simulink model "kh4_controller"  (R2018a)
settings: Solver=ode15s  StartTime=0.0  StopTime=10.0  RelTol=1e-3
libraries: slctrlblks x2, dspinverses x1, simulink x1
settings Model: Creator=FlightControlLab  LastModifiedBy=FlightControlLab
settings SolverCC: SolverResetMethod=Robust

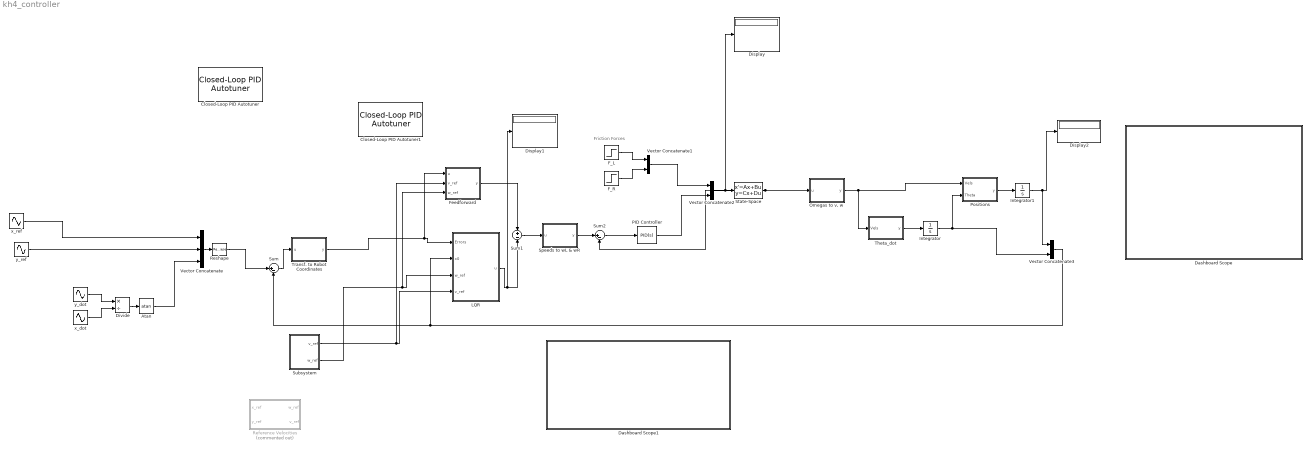
== system kh4_controller ==
  note: Friction Forces
  Atan : Trigonometry  Operator=atan
  Closed-Loop PID Autotuner : slctrlblks/Closed-Loop PID Autotuner  PIDType=PI  PIDForm=Parallel  TimeDomain=continuous-time  DiscreteTs=0.1  IntegratorFormula=Forward Euler  FilterFormula=Forward Euler  ContinuousTs=0.02  Bandwidth=1  UseExternalWC=off  TargetPM=60  UseExternalPM=off  UseExternalAchievedPM=off  PlantType=Stable  PlantSign=Positive  AmpSine=1  UseExternalAmpSine=off  UseExternalFRD=off  UseExternalU0=off  UseCompanion=off  NotDeployTuningModule=off  UsePLCCoder=off  BlockDataType=double  UseConnectedPID=on  blockpath=[]  tunedP=0  tunedI=0  tunedD=0  tunedN=100  tunedPM=0  EstimationWindowSize=3
      settings: SourceProductName=Simulink Control Design  SourceProductBaseCode=SD
  Closed-Loop PID Autotuner1 : slctrlblks/Closed-Loop PID Autotuner  PIDType=PI  PIDForm=Parallel  TimeDomain=discrete-time  DiscreteTs=0.1  IntegratorFormula=Forward Euler  FilterFormula=Forward Euler  ContinuousTs=0.02  Bandwidth=1  UseExternalWC=off  TargetPM=60  UseExternalPM=off  UseExternalAchievedPM=off  PlantType=Stable  PlantSign=Positive  AmpSine=1  UseExternalAmpSine=off  UseExternalFRD=off  UseExternalU0=off  UseCompanion=off  NotDeployTuningModule=off  UsePLCCoder=off  BlockDataType=double  UseConnectedPID=on  blockpath=[]  tunedP=0  tunedI=0  tunedD=0  tunedN=100  tunedPM=0  EstimationWindowSize=3
      settings: SourceProductName=Simulink Control Design  SourceProductBaseCode=SD
  Dashboard Scope : Subsystem  DialogController=hmiCreateDDGDialog  IsWebBlock=on  mask(MWDashboardBlock){webBlockId=dffbf5dc-94e7-4540-87c2-f2341032f13a, webBlockType=sdiscope, ShowInitialText=on, HMISrcModelName=kh4_controller}
      mask prompts: webBlockId "WebBlock Id"; webBlockType "WebBlock Type"; HMISrcModelName "Source Model"
      mask help: SimulinkHMI:dialogs:HMIScopeDialogDesc
      mask Help: helpview([docroot '/mapfiles/simulink.map'], 'hmi_scope')
      mask Display:
      | if strcmp(get_param(bdroot(gcb),'BlockDiagramType'), 'library')
      |     image([(matlabroot) '/toolbox/simulink/hmi/icons/DashboardScope.png']);
      | end
  Dashboard Scope1 : Subsystem  DialogController=hmiCreateDDGDialog  IsWebBlock=on  mask(MWDashboardBlock){webBlockId=52e07cf3-ffb0-4692-b96f-0b5126ad5948, webBlockType=sdiscope, ShowInitialText=on, HMISrcModelName=kh4_controller}
      mask prompts: webBlockId "WebBlock Id"; webBlockType "WebBlock Type"; HMISrcModelName "Source Model"
      mask help: SimulinkHMI:dialogs:HMIScopeDialogDesc
      mask Help: helpview([docroot '/mapfiles/simulink.map'], 'hmi_scope')
      mask Display:
      | if strcmp(get_param(bdroot(gcb),'BlockDiagramType'), 'library')
      |     image([(matlabroot) '/toolbox/simulink/hmi/icons/DashboardScope.png']);
      | end
  Display : Display
  Display1 : Display
  Display2 : Display
  Divide : Product  Inputs=*/
  F_L : Step  After=0.1  SampleTime=0
  F_R : Step  After=0.1  SampleTime=0
  Feedforward : MATLAB Function  TreatAsAtomicUnit=on
  Integrator : Integrator
  Integrator1 : Integrator
  LQR : Subsystem
  "Omegas to v, w" : MATLAB Function  TreatAsAtomicUnit=on
  PID Controller : simulink/Continuous/PID Controller  Controller=PID  TimeDomain=Continuous-time  SampleTime=-1  IntegratorMethod=Forward Euler  FilterMethod=Forward Euler  Form=Parallel  UseFilter=on  ControllerParametersSource=internal  P=10  I=10  D=1  N=100  InitialConditionSource=internal  InitialConditionForIntegrator=0  InitialConditionForFilter=0  ExternalReset=none  LimitOutput=off  UpperSaturationLimit=inf  LowerSaturationLimit=-inf  LinearizeAsGain=on  AntiWindupMode=none  Kb=1  TrackingMode=off  Kt=1  PParamMin=[]  PParamMax=[]  IParamMin=[]  IParamMax=[]  DParamMin=[]  DParamMax=[]  NParamMin=[]  NParamMax=[]  KbParamMin=[]  KbParamMax=[]  KtParamMin=[]  KtParamMax=[]  POutMin=[]  POutMax=[]  IOutMin=[]  IOutMax=[]  DOutMin=[]  DOutMax=[]  NOutMin=[]  NOutMax=[]  KbOutMin=[]  KbOutMax=[]  KtOutMin=[]  KtOutMax=[]  IntegratorOutMin=[]  IntegratorOutMax=[]  FilterOutMin=[]  FilterOutMax=[]  SumOutMin=[]  SumOutMax=[]  SumI1OutMin=[]  SumI1OutMax=[]  SumI2OutMin=[]  SumI2OutMax=[]  SumI3OutMin=[]  SumI3OutMax=[]  SumDOutMin=[]  SumDOutMax=[]  SaturationOutMin=[]  SaturationOutMax=[]  IntegratorContinuousStateAttributes=''  IntegratorStateMustResolveToSignalObject=off  IntegratorRTWStateStorageClass=Auto  FilterContinuousStateAttributes=''  FilterStateMustResolveToSignalObject=off  FilterRTWStateStorageClass=Auto  DifferentiatorICPrevScaledInput=0  DifferentiatorOutMin=[]  DifferentiatorOutMax=[]  FilterDiffOutCoefMin=[]  FilterDiffOutCoefMax=[]  SumDenOutMin=[]  SumDenOutMax=[]  SumNumOutMin=[]  SumNumOutMax=[]  ReciprocalOutMin=[]  ReciprocalOutMax=[]  DivideOutMin=[]  DivideOutMax=[]  TunerSelectOption=Transfer Function Based (PID Tuner App)
  Positions : MATLAB Function  TreatAsAtomicUnit=on
  Reference Velocities : Subsystem  Commented=on
  Reshape : Reshape  OutputDimensionality=Column vector (2-D)
  Speeds to wL & wR : MATLAB Function  TreatAsAtomicUnit=on
  State-Space : StateSpace  A=[0, 0, 0, 0; 0, 0, 0, 0; 0, 0, -0.0100, 0; 0, 0, 0, -0.0100]  B=[1.7699, 1.7699, 0, 0; -0.0072, -0.0072, 0, 0; -0.2100, 0, 0.2100, 0; 0, -0.2100, 0, 10.0000]  C=[0, 0, 1, 0; 0, 0, 0, 1]  D=[0, 0, 0, 0; 0, 0, 0, 0]  InitialCondition=0
  Subsystem : Subsystem
  Sum : Sum  Inputs=|+-
  Sum1 : Sum  Inputs=+-
  Sum2 : Sum  Inputs=|+-
  Theta_dot : MATLAB Function  TreatAsAtomicUnit=on
  Transf. to Robot Coordinates : MATLAB Function  TreatAsAtomicUnit=on
  Vector Concatenate : Concatenate  NumInputs=3
  Vector Concatenate1 : Concatenate
  Vector Concatenate2 : Concatenate
  Vector Concatenate3 : Concatenate
  x_dot : Sin  Amplitude=0.3^2  Frequency=0.3  Phase=pi/2  SampleTime=0
  x_ref : Sin  Amplitude=0.3  Frequency=0.3  SampleTime=0
  y_dot : Sin  Amplitude=-0.3^2  Frequency=0.3  SampleTime=0
  y_ref : Sin  Amplitude=0.3  Frequency=0.3  Phase=pi/2  SampleTime=0
  wires:
  Atan/1 -> Vector Concatenate/3
  x_ref/1 -> Vector Concatenate/1
  y_ref/1 -> Vector Concatenate/2
  Transf. to Robot Coordinates/1(y) -> Feedforward/1(u), LQR/1(Errors)
  Subsystem/2(w_ref) -> Feedforward/3(w_ref), LQR/3(w_ref)
  Sum1/1 -> Speeds to wL & wR/1(u)
  Speeds to wL & wR/1(y) -> Sum2/1
  State-Space/1 -> "Omegas to v, w"/1(u), Sum2/2
  F_L/1 -> Vector Concatenate1/1
  F_R/1 -> Vector Concatenate1/2
  Vector Concatenate2/1 -> Display/1, State-Space/1
  Vector Concatenate1/1 -> Vector Concatenate2/1
  Positions/1(y) -> Integrator1/1
  "Omegas to v, w"/1(y) -> Positions/1(Vels), Theta_dot/1(Vels)
  Theta_dot/1(y) -> Integrator/1
  Integrator/1 -> Vector Concatenate3/2, Positions/2(Theta)
  Integrator1/1 -> Vector Concatenate3/1, Display2/1
  Vector Concatenate3/1 -> Sum/2, LQR/2(x0)
  Subsystem/1(v_ref) -> LQR/4(v_ref), Feedforward/2(v_ref)
  LQR/1(u) -> Sum1/2, Display1/1
  Vector Concatenate/1 -> Reshape/1
  Reshape/1 -> Sum/1
  Sum/1 -> Transf. to Robot Coordinates/1(u)
  Feedforward/1(y) -> Sum1/1
  Divide/1 -> Atan/1
  y_dot/1 -> Divide/1
  x_dot/1 -> Divide/2
  PID Controller/1 -> Vector Concatenate2/2
  Sum2/1 -> PID Controller/1

== system kh4_controller/Dashboard Scope ==

== system kh4_controller/Dashboard Scope1 ==

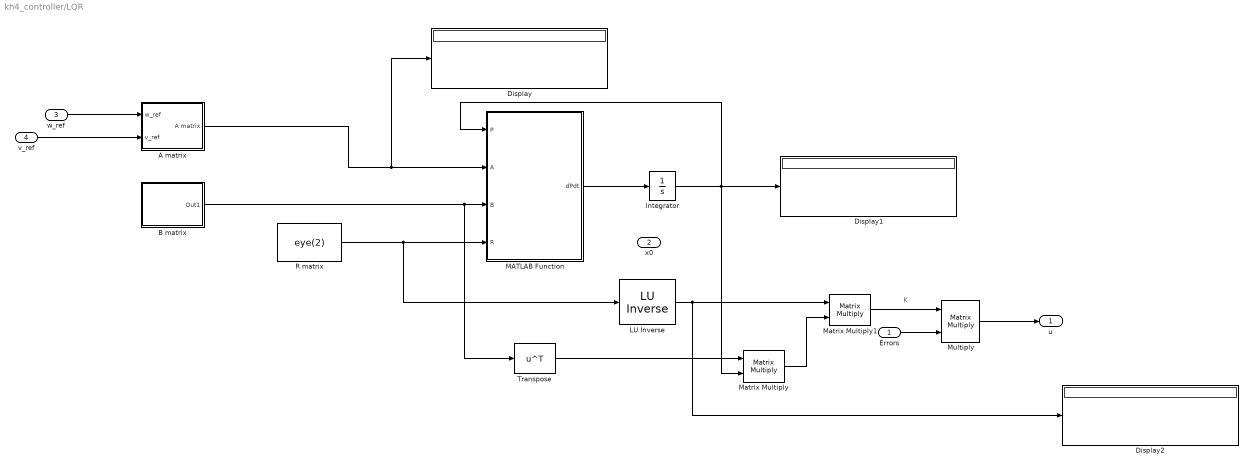
== system kh4_controller/LQR ==
  note: K
  Errors : Inport
  x0 : Inport  Port=2
  w_ref : Inport  Port=3
  v_ref : Inport  Port=4
  " LU Inverse" : dspinverses/ LU Inverse
      settings: SourceProductName=DSP System Toolbox
  A matrix : Subsystem
  B matrix : Subsystem
  Display : Display
  Display1 : Display
  Display2 : Display
  Integrator : Integrator  InitialCondition=ones(3,3)
  MATLAB Function : MATLAB Function  TreatAsAtomicUnit=on
  Matrix Multiply : Product  Multiplication=Matrix(*)
  Matrix Multiply1 : Product  Multiplication=Matrix(*)
  Multiply : Product  Multiplication=Matrix(*)
  R matrix : Constant  Value=eye(2)  VectorParams1D=off
  Transpose : Math  Operator=transpose  SaturateOnIntegerOverflow=on
  u : Outport
  wires:
  B matrix/1(Out1) -> Transpose/1, MATLAB Function/3(B)
  Matrix Multiply1/1 -> Multiply/1
  R matrix/1 -> " LU Inverse"/1, MATLAB Function/4(R)
  A matrix/1(A matrix) -> Display/1, MATLAB Function/2(A)
  Multiply/1 -> u/1
  Integrator/1 -> MATLAB Function/1(P), Display1/1, Matrix Multiply/2
  Matrix Multiply/1 -> Matrix Multiply1/2
  Transpose/1 -> Matrix Multiply/1
  MATLAB Function/1(dPdt) -> Integrator/1
  w_ref/1 -> A matrix/1(w_ref)
  v_ref/1 -> A matrix/2(v_ref)
  " LU Inverse"/1 -> Display2/1, Matrix Multiply1/1
  Errors/1 -> Multiply/2

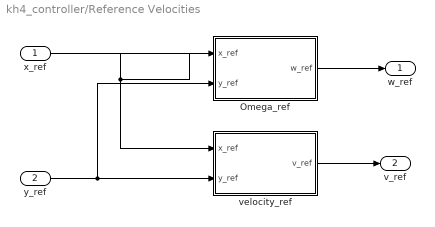
== system kh4_controller/Reference Velocities ==
  x_ref : Inport
  y_ref : Inport  Port=2
  Omega_ref : Subsystem
  velocity_ref : Subsystem
  w_ref : Outport
  v_ref : Outport  Port=2
  wires:
  y_ref/1 -> Omega_ref/2(y_ref), velocity_ref/2(y_ref)
  Omega_ref/1(w_ref) -> w_ref/1
  velocity_ref/1(v_ref) -> v_ref/1
  x_ref/1 -> Omega_ref/1(x_ref), velocity_ref/1(x_ref)

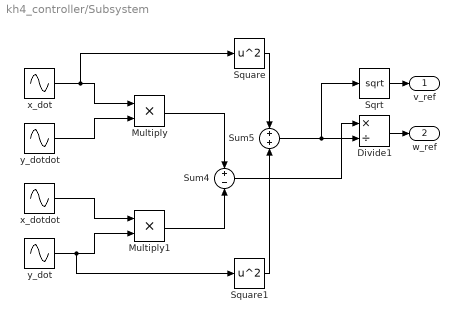
== system kh4_controller/Subsystem ==
  Divide1 : Product  Inputs=*/
  Multiply : Product
  Multiply1 : Product
  Sqrt : Sqrt  SaturateOnIntegerOverflow=on
  Square : Math  Operator=square  SaturateOnIntegerOverflow=on
  Square1 : Math  Operator=square  SaturateOnIntegerOverflow=on
  Sum4 : Sum  Inputs=+-
  Sum5 : Sum
  x_dot : Sin  Amplitude=0.3^2  Frequency=0.3  Phase=pi/2  SampleTime=0
  x_dotdot : Sin  Amplitude=-0.3^3  Frequency=0.3  SampleTime=0
  y_dot : Sin  Amplitude=-0.3^2  Frequency=0.3  SampleTime=0
  y_dotdot : Sin  Amplitude=-0.3^3  Frequency=0.3  Phase=pi/2  SampleTime=0
  v_ref : Outport
  w_ref : Outport  Port=2
  wires:
  x_dot/1 -> Square/1, Multiply/1
  Divide1/1 -> w_ref/1
  x_dotdot/1 -> Multiply1/1
  Sum5/1 -> Divide1/2, Sqrt/1
  Square/1 -> Sum5/1
  Sum4/1 -> Divide1/1
  y_dot/1 -> Square1/1, Multiply1/2
  y_dotdot/1 -> Multiply/2
  Multiply1/1 -> Sum4/2
  Square1/1 -> Sum5/2
  Multiply/1 -> Sum4/1
  Sqrt/1 -> v_ref/1

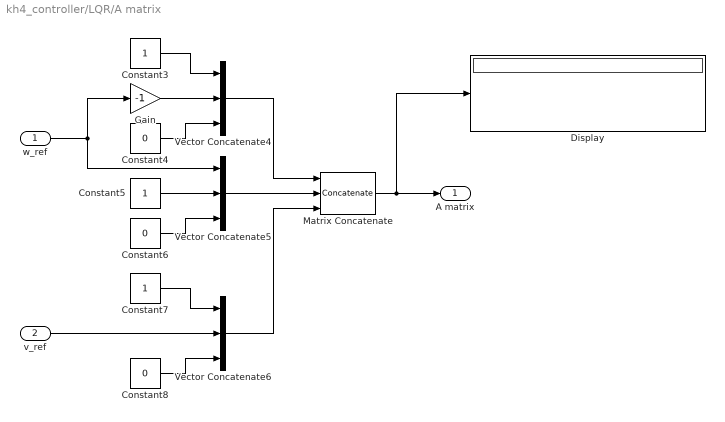
== system kh4_controller/LQR/A matrix ==
  w_ref : Inport
  v_ref : Inport  Port=2
  Constant3 : Constant
  Constant4 : Constant  Value=0
  Constant5 : Constant
  Constant6 : Constant  Value=0
  Constant7 : Constant
  Constant8 : Constant  Value=0
  Display : Display
  Gain : Gain  Gain=-1
  Matrix Concatenate : Concatenate  NumInputs=3  Mode=Multidimensional array  ConcatenateDimension=2
  Vector Concatenate4 : Concatenate  NumInputs=3
  Vector Concatenate5 : Concatenate  NumInputs=3
  Vector Concatenate6 : Concatenate  NumInputs=3
  A matrix : Outport
  wires:
  w_ref/1 -> Gain/1, Vector Concatenate5/1
  Gain/1 -> Vector Concatenate4/2
  Constant6/1 -> Vector Concatenate5/3
  Vector Concatenate6/1 -> Matrix Concatenate/3
  Constant4/1 -> Vector Concatenate4/3
  v_ref/1 -> Vector Concatenate6/2
  Constant7/1 -> Vector Concatenate6/1
  Vector Concatenate5/1 -> Matrix Concatenate/2
  Constant8/1 -> Vector Concatenate6/3
  Constant3/1 -> Vector Concatenate4/1
  Constant5/1 -> Vector Concatenate5/2
  Vector Concatenate4/1 -> Matrix Concatenate/1
  Matrix Concatenate/1 -> Display/1, A matrix/1

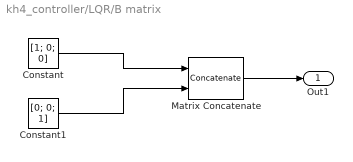
== system kh4_controller/LQR/B matrix ==
  Constant : Constant  Value=[1; 0; 0]  VectorParams1D=off
  Constant1 : Constant  Value=[0; 0; 1]  VectorParams1D=off
  Matrix Concatenate : Concatenate  Mode=Multidimensional array  ConcatenateDimension=2
  Out1 : Outport
  wires:
  Constant/1 -> Matrix Concatenate/1
  Matrix Concatenate/1 -> Out1/1
  Constant1/1 -> Matrix Concatenate/2

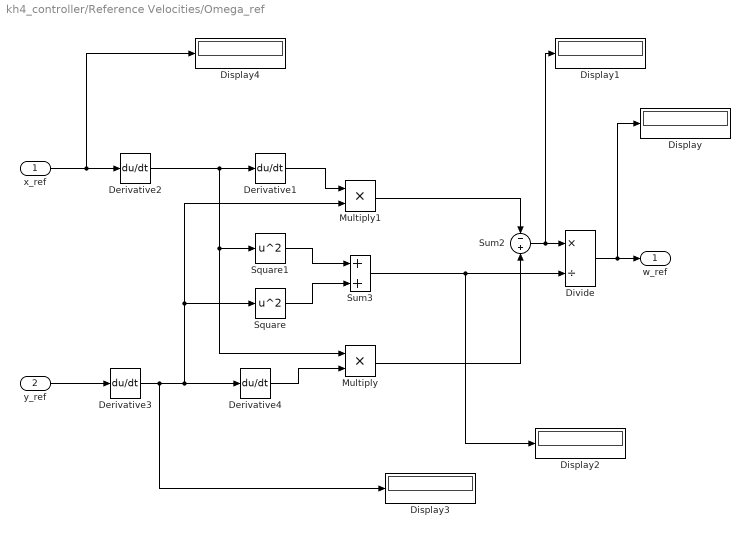
== system kh4_controller/Reference Velocities/Omega_ref ==
  x_ref : Inport
  y_ref : Inport  Port=2
  Derivative{1..4} (4 alike) : Derivative  CoefficientInTFapproximation=1
  Display{,1..4} (5 alike) : Display
  Divide : Product  Inputs=*/
  Multiply : Product
  Multiply1 : Product  InputSameDT=on
  Square : Math  Operator=square  SaturateOnIntegerOverflow=on
  Square1 : Math  Operator=square  SaturateOnIntegerOverflow=on
  Sum2 : Sum  Inputs=-+
  Sum3 : Sum
  w_ref : Outport
  wires:
  Square/1 -> Sum3/2
  Sum3/1 -> Divide/2, Display2/1
  Sum2/1 -> Display1/1, Divide/1
  Derivative3/1 -> Display3/1, Derivative4/1, Square/1, Multiply1/2
  Square1/1 -> Sum3/1
  Divide/1 -> Display/1, w_ref/1
  Multiply1/1 -> Sum2/1
  Multiply/1 -> Sum2/2
  Derivative4/1 -> Multiply/2
  x_ref/1 -> Display4/1, Derivative2/1
  Derivative1/1 -> Multiply1/1
  y_ref/1 -> Derivative3/1
  Derivative2/1 -> Derivative1/1, Multiply/1, Square1/1

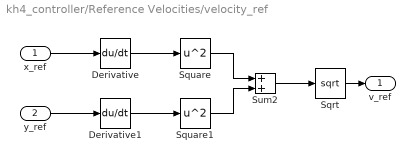
== system kh4_controller/Reference Velocities/velocity_ref ==
  x_ref : Inport
  y_ref : Inport  Port=2
  Derivative : Derivative
  Derivative1 : Derivative
  Sqrt : Sqrt  SaturateOnIntegerOverflow=on
  Square : Math  Operator=square  SaturateOnIntegerOverflow=on
  Square1 : Math  Operator=square  SaturateOnIntegerOverflow=on
  Sum2 : Sum
  v_ref : Outport
  wires:
  Square/1 -> Sum2/1
  Sum2/1 -> Sqrt/1
  Derivative/1 -> Square/1
  Sqrt/1 -> v_ref/1
  Derivative1/1 -> Square1/1
  Square1/1 -> Sum2/2
  y_ref/1 -> Derivative1/1
  x_ref/1 -> Derivative/1

== matlab function kh4_controller/Transf. to Robot Coordinates ==
  data: u input size=[3,1]; y output size=[3,1]
function y = fcn(u)

theta = u(3);
A = [cosd(theta), sind(theta), 0;
    -sind(theta), cosd(theta), 0;
    0, 0, 1];

y = A*u;

== matlab function kh4_controller/Feedforward ==
  data: u input size=[3,1]; y output size=[2,1]; v_ref input size=1; w_ref input size=1
function y = fcn(u, v_ref, w_ref)

    e3 = u(3);
    
    y = [cos(e3)*v_ref;
        w_ref];

== matlab function kh4_controller/Speeds to wL & wR ==
  data: u input size=2; y output size=2
function y = fcn(u)

r = 0.021; % Wheel radius
D = 0.145; % Robot diameter

v = u(1);
w = u(2);

v_r = (2*v+w*D)/2;
v_l = (2*v-w*D)/2;

w_l = v_l/r;
w_r = v_r/r;

y =  [w_l;
    w_r];

== matlab function kh4_controller/Theta_dot ==
  data: Vels input size=2; y output size=1
function y = fcn(Vels)

y = Vels(2);

== matlab function kh4_controller/Positions ==
  data: Vels input size=2; Theta input size=1; y output size=2
function y = fcn(Vels, Theta)

v = Vels(1);

x1 = v * cosd(Theta);
x2 = v * sind(Theta);

y = [x1; x2];

== matlab function kh4_controller/Omegas to v, w ==
  data: u input size=2; y output size=2
function y = fcn(u)
r = 0.021; % Wheel radius
D = 0.145; % Robot diameter

v = u*r; 

v_l = v(1);
v_r = v(2);

omega = (v_r - v_l)/D;
v = (v_r + v_l)/2;

y = [v; omega];

== matlab function kh4_controller/LQR/MATLAB Function ==
  data: dPdt output size=[3,3]; P input size=[3,3]; A input size=[3,3]; B input size=[3,2]; R input size=[2,2]
function dPdt  = mRiccati(P,A,B,R)

% A = rand(3,3);
% B = rand(3,2);
Q = diag([1 1 10]);
% R = 1e-4*diag([1 1]);
% P = rand(3,3);

% Continuous Riccati differential equation
dPdt = -(A'*P + P*A - (P*B)*pinv(R)*(B'*P) + Q);
